simulink model "sm_car_test_ggv_new"  (R2026a)
settings: Solver=ode23t  StopTime=300  MaxStep=0.4  AbsTol=1e-3  EnableMultiTasking=on
PreLoadFcn:
  | % PreLoadFcn Removed for GGV Sweep
PostLoadFcn:
  | % PostLoadFcn Removed for GGV Sweep
InitFcn:
  | sm_car_config_camera;
  | Vehicle = sm_car_vehcfg_checkConfig(Vehicle);
  | sm_car_check_tire_model(bdroot);
StartFcn:
  | tic;
StopFcn:
  | Elapsed_Sim_Time = toc;
  | % disp(['Elapsed Sim Time = ' num2str(Elapsed_Sim_Time)]);
values from neighbouring files (symbols this model uses):
  accel_ramp_rate = 0.1    [sm_car_sweep_ggv_pts.m]
undefined symbols (not defined in the file or in its folder): acc_theta, Axle1D, AxleIn, Camera, Control, drag_frc, Driver, Init, lift_frc, Maneuver, Pedal, Scene, ShaftL1, ShaftL2, ShaftR1, ShaftR2, Visual, X, xy_data_car_side, Y, Z
libraries: sm_lib x270, fl_lib x171, nesl_utility x137, simulink x56, sdl_lib x14, simulink_extras x11, SimscapeFluids_lib x7, Scene_Utilities x6, dspsigops x4, Damper_Element x4, Tire_1x2x x4, ee_lib x3
(part 10 of 20)

== system sm_car_test_ggv_new/World/Scene/Skidpad/Circle Outer L ==
  Solid : sm_lib/Body Elements/Extruded Solid  ExtrusionType=General  PolygonNumSides=3  PolygonOuterRadius=1  PolygonOuterRadiusUnits=m  ExportEntireGeometry=off  ExtrusionCrossSection=xy_data_circ  ExtrusionCrossSectionUnits=m  ExportConvexHullGeometry=off  ExtrusionLength=circ_h  ExtrusionLengthUnits=m  InertiaType=CalculateFromGeometry  BasedOnType=Density  Density=1000  DensityUnits=kg/m^3  Mass=1  MassUnits=kg  CenterOfMass=[0 0 0]  CenterOfMassUnits=m  MomentsOfInertia=[1 1 1]  MomentsOfInertiaUnits=kg*m^2  ProductsOfInertia=[1 1 1]  ProductsOfInertiaUnits=kg*m^2  GraphicType=FromGeometry  MarkerShape=Sphere  MarkerSize=10  GraphicVisPropType=SimpleVisualProperties  GraphicDiffuseColor=[1.0 1.0 0.8]  GraphicOpacity=1.0  GraphicSpecularColor=[0.5 0.5 0.5 1.0]  GraphicAmbientColor=[0.15 0.15 0.15 1.0]  GraphicEmissiveColor=[0.0 0.0 0.0 1.0]  GraphicShininess=75  DoExposeReferenceFrame=on  SerializedFrames=<Frames/>
  W : PMIOPort  Side=Right
  connections:
  Solid/RConn1 -- W/RConn1

== system sm_car_test_ggv_new/World/Scene/Skidpad/Circle Outer R ==
  Solid : sm_lib/Body Elements/Extruded Solid  ExtrusionType=General  PolygonNumSides=3  PolygonOuterRadius=1  PolygonOuterRadiusUnits=m  ExportEntireGeometry=off  ExtrusionCrossSection=xy_data_circ  ExtrusionCrossSectionUnits=m  ExportConvexHullGeometry=off  ExtrusionLength=circ_h  ExtrusionLengthUnits=m  InertiaType=CalculateFromGeometry  BasedOnType=Density  Density=1000  DensityUnits=kg/m^3  Mass=1  MassUnits=kg  CenterOfMass=[0 0 0]  CenterOfMassUnits=m  MomentsOfInertia=[1 1 1]  MomentsOfInertiaUnits=kg*m^2  ProductsOfInertia=[1 1 1]  ProductsOfInertiaUnits=kg*m^2  GraphicType=FromGeometry  MarkerShape=Sphere  MarkerSize=10  GraphicVisPropType=SimpleVisualProperties  GraphicDiffuseColor=[1.0 1.0 0.8]  GraphicOpacity=1.0  GraphicSpecularColor=[0.5 0.5 0.5 1.0]  GraphicAmbientColor=[0.15 0.15 0.15 1.0]  GraphicEmissiveColor=[0.0 0.0 0.0 1.0]  GraphicShininess=75  DoExposeReferenceFrame=on  SerializedFrames=<Frames/>
  W : PMIOPort  Side=Right
  connections:
  Solid/RConn1 -- W/RConn1

== system sm_car_test_ggv_new/World/Scene/Skidpad/Ground Plane ==
  Floor : sm_lib/Body Elements/Brick Solid  BrickDimensions=[gp_l, gp_w, gp_h]  BrickDimensionsUnits=m  ExportEntireGeometry=off  InertiaType=CalculateFromGeometry  BasedOnType=Density  Density=1000  DensityUnits=kg/m^3  Mass=1  MassUnits=kg  CenterOfMass=[0 0 0]  CenterOfMassUnits=m  MomentsOfInertia=[1 1 1]  MomentsOfInertiaUnits=kg*m^2  ProductsOfInertia=[0 0 0]  ProductsOfInertiaUnits=kg*m^2  GraphicType=FromGeometry  MarkerShape=Sphere  MarkerSize=10  GraphicVisPropType=SimpleVisualProperties  GraphicDiffuseColor=gp_clr  GraphicOpacity=gp_opc  GraphicSpecularColor=[0.5 0.5 0.5 1.0]  GraphicAmbientColor=[0.15 0.15 0.15 1.0]  GraphicEmissiveColor=[0.0 0.0 0.0 1.0]  GraphicShininess=75  DoExposeReferenceFrame=off  SerializedFrames=<Frames><Frame><Id>Frame1</Id><Value><Name>F</Name><Origin><Source>GeometricFeature</Source><FeatureName>+z surface</FeatureName></Origin><PrimaryAxis><DefinedDirection>+Z</DefinedDirection><Source>ReferenceFrame</Source><SourceDirection>+Z</SourceDirection><FeatureName></FeatureName></PrimaryAxis><SecondaryAxis><DefinedDirection>+X</DefinedDirection><Source>ReferenceFrame</Source><SourceDirection>+X</SourceDirection><FeatureName></FeatureName></SecondaryAxis></Value></Frame></Frames>
  W : PMIOPort  Side=Right
  connections:
  Floor/LConn1 -- W/RConn1

== system sm_car_test_ggv_new/Controller/Default/State Estimation/Sensor Noise Simulation/noise COG ==
  <vx> : Inport
  <COG> : Inport  Port=2
  Add1 : Sum
  Add2 : Sum
  Band-Limited White Noise1 : simulink/Sources/Band-Limited White Noise  Cov=[7e-3]  Ts=0.1  seed=[08854]
  Band-Limited White Noise2 : simulink/Sources/Band-Limited White Noise  Cov=[1.2e-5]  Ts=0.1  seed=[08854]
  Compare To Constant : simulink/Logic and Bit Operations/Compare To Constant  relop=<=  const=0.15  OutDataTypeStr=boolean
  Quantizer1 : Quantizer  QuantizationInterval=deg2rad(0.1)
  Quantizer2 : Quantizer  QuantizationInterval=deg2rad(0.1)
  Switch : Switch  Criteria=u2 ~= 0  SaturateOnIntegerOverflow=off  InputSameDT=off
  Zero-Order Hold1 : ZeroOrderHold  SampleTime=0.1
  Zero-Order Hold2 : ZeroOrderHold  SampleTime=0.1
  COG_n : Outport
  wires:
  Add2/1 -> Switch/3  "COG_n"
  <COG>/1 -> Quantizer1/1, Quantizer2/1
  Zero-Order Hold2/1 -> Add2/1
  Band-Limited White Noise2/1 -> Add2/2
  Quantizer2/1 -> Zero-Order Hold2/1
  <vx>/1 -> Compare To Constant/1
  Compare To Constant/1 -> Switch/2
  Quantizer1/1 -> Zero-Order Hold1/1
  Band-Limited White Noise1/1 -> Add1/2
  Zero-Order Hold1/1 -> Add1/1
  Add1/1 -> Switch/1  "COG_n"
  Switch/1 -> COG_n/1

== system sm_car_test_ggv_new/Controller/Default/State Estimation/Sensor Noise Simulation/noise a_x ==
  <w> : Inport
  Add2 : Sum
  Band-Limited White Noise2 : simulink/Sources/Band-Limited White Noise  Cov=[0.0024]  Ts=0.01  seed=[512361]
  Quantizer2 : Quantizer  QuantizationInterval=0.0047
  Zero-Order Hold2 : ZeroOrderHold  SampleTime=0.01
  a_x_n : Outport
  wires:
  Add2/1 -> a_x_n/1  "a_x_n"
  <w>/1 -> Quantizer2/1
  Zero-Order Hold2/1 -> Add2/1
  Band-Limited White Noise2/1 -> Add2/2
  Quantizer2/1 -> Zero-Order Hold2/1

== system sm_car_test_ggv_new/Controller/Default/State Estimation/Sensor Noise Simulation/noise a_y ==
  <w> : Inport
  Add2 : Sum
  Band-Limited White Noise2 : simulink/Sources/Band-Limited White Noise  Cov=[0.0024]  Ts=0.01  seed=[092756]
  Quantizer2 : Quantizer  QuantizationInterval=0.0047
  Zero-Order Hold2 : ZeroOrderHold  SampleTime=0.01
  a_y_n : Outport
  wires:
  Add2/1 -> a_y_n/1  "a_y_n"
  <w>/1 -> Quantizer2/1
  Zero-Order Hold2/1 -> Add2/1
  Band-Limited White Noise2/1 -> Add2/2
  Quantizer2/1 -> Zero-Order Hold2/1

== system sm_car_test_ggv_new/Controller/Default/State Estimation/Sensor Noise Simulation/noise omega_fl ==
  <w> : Inport
  Add2 : Sum
  Band-Limited White Noise2 : simulink/Sources/Band-Limited White Noise  Cov=[1e-4]  Ts=0.01  seed=[12451]
  Quantizer2 : Quantizer  QuantizationInterval=2 * pi / 25
  Zero-Order Hold2 : ZeroOrderHold  SampleTime=0.01
  omega_rl : Outport
  wires:
  Add2/1 -> omega_rl/1  "omega_rl"
  <w>/1 -> Quantizer2/1
  Zero-Order Hold2/1 -> Add2/1
  Band-Limited White Noise2/1 -> Add2/2
  Quantizer2/1 -> Zero-Order Hold2/1

== system sm_car_test_ggv_new/Controller/Default/State Estimation/Sensor Noise Simulation/noise omega_fr ==
  <w> : Inport
  Add3 : Sum
  Band-Limited White Noise3 : simulink/Sources/Band-Limited White Noise  Cov=[1e-4]  Ts=0.01  seed=[68595]
  Quantizer3 : Quantizer  QuantizationInterval=2 * pi / 25
  Zero-Order Hold3 : ZeroOrderHold  SampleTime=0.01
  omega_rr : Outport
  wires:
  Add3/1 -> omega_rr/1  "omega_rr"
  Band-Limited White Noise3/1 -> Add3/2
  Zero-Order Hold3/1 -> Add3/1
  <w>/1 -> Quantizer3/1
  Quantizer3/1 -> Zero-Order Hold3/1

== system sm_car_test_ggv_new/Controller/Default/State Estimation/Sensor Noise Simulation/noise omega_rl ==
  <w> : Inport
  Add : Sum
  Band-Limited White Noise : simulink/Sources/Band-Limited White Noise  Cov=[1e-4]  Ts=0.01  seed=[23341]
  Quantizer : Quantizer  QuantizationInterval=2 * pi / 94
  Zero-Order Hold : ZeroOrderHold  SampleTime=0.01
  omega_rl : Outport
  wires:
  Quantizer/1 -> Zero-Order Hold/1
  <w>/1 -> Quantizer/1
  Band-Limited White Noise/1 -> Add/2
  Add/1 -> omega_rl/1  "omega_rl"
  Zero-Order Hold/1 -> Add/1

== system sm_car_test_ggv_new/Controller/Default/State Estimation/Sensor Noise Simulation/noise omega_rr ==
  <w> : Inport
  Add1 : Sum
  Band-Limited White Noise1 : simulink/Sources/Band-Limited White Noise  Cov=[1e-4]  Ts=0.01  seed=[41245]
  Quantizer1 : Quantizer  QuantizationInterval=2 * pi / 94
  Zero-Order Hold1 : ZeroOrderHold  SampleTime=0.01
  omega_rr : Outport
  wires:
  Add1/1 -> omega_rr/1  "omega_rr"
  Quantizer1/1 -> Zero-Order Hold1/1
  <w>/1 -> Quantizer1/1
  Band-Limited White Noise1/1 -> Add1/2
  Zero-Order Hold1/1 -> Add1/1

== system sm_car_test_ggv_new/Controller/Default/State Estimation/Sensor Noise Simulation/noise v_gps ==
  <vz> : Inport
  <vx> : Inport  Port=2
  <vy> : Inport  Port=3
  Add : Sum  Inputs=+++
  Add2 : Sum
  Band-Limited White Noise2 : simulink/Sources/Band-Limited White Noise  Cov=[9e-4]  Ts=0.1  seed=[645743]
  Quantizer2 : Quantizer  QuantizationInterval=0.01
  Sqrt : Sqrt
  Square : Math  Operator=square
  Square1 : Math  Operator=square
  Square2 : Math  Operator=square
  Zero-Order Hold2 : ZeroOrderHold  SampleTime=0.1
  V_GPS_n : Outport
  wires:
  Quantizer2/1 -> Zero-Order Hold2/1
  Band-Limited White Noise2/1 -> Add2/2
  Zero-Order Hold2/1 -> Add2/1
  Sqrt/1 -> Quantizer2/1
  Add2/1 -> V_GPS_n/1  "V_GPS_n"
  <vz>/1 -> Square/1
  <vx>/1 -> Square1/1
  <vy>/1 -> Square2/1
  Add/1 -> Sqrt/1
  Square/1 -> Add/1
  Square1/1 -> Add/2
  Square2/1 -> Add/3

== system sm_car_test_ggv_new/Controller/Default/State Estimation/Sensor Noise Simulation/noise yaw ==
  <w> : Inport
  Add2 : Sum
  Band-Limited White Noise2 : simulink/Sources/Band-Limited White Noise  Cov=[1.2e-7]  Ts=0.01  seed=[211845]
  Quantizer2 : Quantizer  QuantizationInterval=deg2rad(0.1)
  Zero-Order Hold2 : ZeroOrderHold  SampleTime=0.01
  aYaw_n : Outport
  wires:
  Quantizer2/1 -> Zero-Order Hold2/1
  Band-Limited White Noise2/1 -> Add2/2
  Zero-Order Hold2/1 -> Add2/1
  <w>/1 -> Quantizer2/1
  Add2/1 -> aYaw_n/1  "aYaw_n"

== system sm_car_test_ggv_new/Controller/Default/State Estimation/Sensor Noise Simulation/noise yaw rate ==
  <w> : Inport
  Add2 : Sum
  Band-Limited White Noise2 : simulink/Sources/Band-Limited White Noise  Cov=[7.6e-7]  Ts=0.01  seed=[809953]
  Quantizer2 : Quantizer  QuantizationInterval=0.001
  Zero-Order Hold2 : ZeroOrderHold  SampleTime=0.01
  nYaw_n : Outport
  wires:
  Quantizer2/1 -> Zero-Order Hold2/1
  Band-Limited White Noise2/1 -> Add2/2
  Zero-Order Hold2/1 -> Add2/1
  <w>/1 -> Quantizer2/1
  Add2/1 -> nYaw_n/1  "nYaw_n"

== system sm_car_test_ggv_new/Controller/TrqVec 4Motor/Brake Control/ABS/Calculate Slip ==
  WhlSpd : Inport
  VehSpdEst : Inport  Port=2
  Abs : Abs  ZeroCross=off  SaturateOnIntegerOverflow=off
  Bus Creator : BusCreator  Inputs=4
  Bus Selector1 : BusSelector  OutputSignals=L1.v,R1.v,L2.v,R2.v
  Constant : Constant
  Demux : Demux
  Fcn{,1..3} (4 alike) : Fcn  Expr=abs(u(1)*u(2)-u(3))/u(3)
  Mux{,1..3} (4 alike) : Mux  Inputs=3
  Mux4 : Mux
  Mux5 : Mux
  Product : Product
  Saturation : Saturate  UpperLimit=inf  LowerLimit=eps  ZeroCross=off
  Saturation1 : Saturate  UpperLimit=1  LowerLimit=0
  Sign : Signum  ZeroCross=off
  Wheel Speeds and Slip : Scope  NumInputPorts=2
      settings: ActiveDisplayYMinimum=-11.64241  ActiveDisplayYMaximum=114.01232  DataLoggingVariableName=ScopeData2
  Slip : Outport  VectorParamsAs1DForOutWhenUnconnected=off
  wires:
  WhlSpd/1 -> Bus Selector1/1
  Bus Selector1/2 -> Mux4/2, Mux1/2  "<v>"
  Bus Selector1/4 -> Mux4/4, Mux3/2  "<v>"
  Bus Selector1/1 -> Mux4/1, Mux/2  "<v>"
  Bus Selector1/3 -> Mux4/3, Mux2/2  "<v>"
  Constant/1 -> Mux/1, Mux1/1, Mux3/1, Mux2/1
  VehSpdEst/1 -> Sign/1, Abs/1
  Demux/1 -> Bus Creator/1  "L1"
  Demux/2 -> Bus Creator/2  "R1"
  Demux/3 -> Bus Creator/3  "L2"
  Demux/4 -> Bus Creator/4  "R2"
  Bus Creator/1 -> Wheel Speeds and Slip/2, Slip/1  "Slip"
  Product/1 -> Mux3/3, Mux2/3, Mux1/3, Mux/3
  Abs/1 -> Saturation/1
  Saturation/1 -> Product/1
  Sign/1 -> Product/2
  Mux/1 -> Fcn/1
  Mux1/1 -> Fcn1/1
  Mux2/1 -> Fcn2/1
  Mux3/1 -> Fcn3/1
  Mux4/1 -> Wheel Speeds and Slip/1  "Wheel Speeds"
  Mux5/1 -> Saturation1/1
  Saturation1/1 -> Demux/1
  Fcn/1 -> Mux5/1  "L1"
  Fcn1/1 -> Mux5/2  "R1"
  Fcn2/1 -> Mux5/3  "L2"
  Fcn3/1 -> Mux5/4  "R2"

== system sm_car_test_ggv_new/Controller/TrqVec 4Motor/Brake Control/ABS/Sensor ==
  Body : Inport
  WhlSpd : Inport  Port=2
  Bus Creator{,3..5} (4 alike) : BusCreator  Inputs=1
  Bus Creator6 : BusCreator  Inputs=5
  Bus Selector : BusSelector  OutputSignals=vx,vy  OutputAsBus=on
  Bus Selector4 : BusSelector  OutputSignals=WhlL1.n,WhlR1.n,WhlL2.n,WhlR2.n,WhlL2.qxyz
  Gain : Gain  Gain=3.6*abs_tire_radiusF
  Gain1 : Gain  Gain=3.6*abs_tire_radiusF
  Gain2 : Gain  Gain=3.6*abs_tire_radiusR
  Gain3 : Gain  Gain=3.6*abs_tire_radiusR
  Gain4 : Gain  Gain=3.6
  Terminator1 : Terminator  Commented=on
  Vel in xy plane : Fcn  Expr=sqrt(u(1)^2+u(2)^2)
  missing tooth : Subsystem  Commented=on
  GroundSpd : Outport  VectorParamsAs1DForOutWhenUnconnected=off
  wires:
  Gain1/1 -> Bus Creator3/1  "v"
  missing tooth/1(Out1) -> Terminator1/1  "v"
  Gain2/1 -> Bus Creator4/1  "v"
  Bus Selector4/5 -> missing tooth/2(<qxyz>)  "<qxyz>"
  Bus Creator5/1 -> Bus Creator6/5  "R2"
  Gain3/1 -> Bus Creator5/1  "v"
  Bus Creator/1 -> Bus Creator6/2  "L1"
  Bus Selector4/2 -> Gain1/1  "<n>"
  Bus Creator4/1 -> Bus Creator6/4  "L2"
  Bus Selector4/3 -> Gain2/1, missing tooth/1(<omega>)  "<n>"
  Gain/1 -> Bus Creator/1  "v"
  Body/1 -> Bus Selector/1
  Bus Creator3/1 -> Bus Creator6/3  "R1"
  Gain4/1 -> Bus Creator6/1  "v"
  Bus Selector4/1 -> Gain/1  "<n>"
  Bus Selector4/4 -> Gain3/1  "<n>"
  WhlSpd/1 -> Bus Selector4/1
  Bus Creator6/1 -> GroundSpd/1
  Vel in xy plane/1 -> Gain4/1  "speed"
  Bus Selector/1 -> Vel in xy plane/1

== system sm_car_test_ggv_new/Controller/TrqVec 4Motor/Brake Control/ABS/Valve Control L1 ==
  Slip : Inport
  vSpdEst : Inport  Port=2
  Categorize Surface : Subsystem
  Code to Valves : Subsystem
  Demux : Demux  Outputs=2
  Logic : Stateflow chart  TreatAsAtomicUnit=on
  Mux : Mux  Inputs=2
  Product : Product
  Subsystem : Subsystem
  Subsystem1 : Subsystem
  Valve : Outport  VectorParamsAs1DForOutWhenUnconnected=off
  wires:
  Logic/1(Mod_State) -> Categorize Surface/1(Mod State), Code to Valves/1(C)
  Logic/2(Mod_Dur) -> Product/2
  Slip/1 -> Logic/1(Slip)
  Code to Valves/1(V) -> Product/1
  vSpdEst/1 -> Logic/2(vSpdEst)
  Product/1 -> Demux/1
  Demux/1 -> Subsystem/1(OnT)
  Demux/2 -> Subsystem1/1(OnT)
  Mux/1 -> Valve/1
  Subsystem/1(vSig) -> Mux/1, Categorize Surface/2(Apply Valve)
  Subsystem1/1(vSig) -> Mux/2

== system sm_car_test_ggv_new/Controller/TrqVec 4Motor/Brake Control/ABS/Valve Control L2 ==
  Slip : Inport
  vSpdEst : Inport  Port=2
  Categorize Surface : Subsystem
  Code to Valves : Subsystem
  Demux : Demux  Outputs=2
  Logic : Stateflow chart  TreatAsAtomicUnit=on
  Mux : Mux  Inputs=2
  Product : Product
  Subsystem : Subsystem
  Subsystem1 : Subsystem
  Valve : Outport  VectorParamsAs1DForOutWhenUnconnected=off
  wires:
  Logic/1(Mod_State) -> Categorize Surface/1(Mod State), Code to Valves/1(C)
  Logic/2(Mod_Dur) -> Product/2
  Slip/1 -> Logic/1(Slip)
  Code to Valves/1(V) -> Product/1
  vSpdEst/1 -> Logic/2(vSpdEst)
  Product/1 -> Demux/1
  Demux/1 -> Subsystem/1(OnT)
  Demux/2 -> Subsystem1/1(OnT)
  Mux/1 -> Valve/1
  Subsystem/1(vSig) -> Mux/1, Categorize Surface/2(Apply Valve)
  Subsystem1/1(vSig) -> Mux/2

== system sm_car_test_ggv_new/Controller/TrqVec 4Motor/Brake Control/ABS/Valve Control R1 ==
  Slip : Inport
  vSpdEst : Inport  Port=2
  Categorize Surface : Subsystem
  Code to Valves : Subsystem
  Demux : Demux  Outputs=2
  Logic : Stateflow chart  TreatAsAtomicUnit=on
  Mux : Mux  Inputs=2
  Product : Product
  Subsystem : Subsystem
  Subsystem1 : Subsystem
  Valve : Outport  VectorParamsAs1DForOutWhenUnconnected=off
  wires:
  Logic/1(Mod_State) -> Categorize Surface/1(Mod State), Code to Valves/1(C)
  Logic/2(Mod_Dur) -> Product/2
  Slip/1 -> Logic/1(Slip)
  Code to Valves/1(V) -> Product/1
  vSpdEst/1 -> Logic/2(vSpdEst)
  Product/1 -> Demux/1
  Demux/1 -> Subsystem/1(OnT)
  Demux/2 -> Subsystem1/1(OnT)
  Mux/1 -> Valve/1
  Subsystem/1(vSig) -> Mux/1, Categorize Surface/2(Apply Valve)
  Subsystem1/1(vSig) -> Mux/2

== system sm_car_test_ggv_new/Controller/TrqVec 4Motor/Brake Control/ABS/Valve Control R2 ==
  Slip : Inport
  vSpdEst : Inport  Port=2
  Categorize Surface : Subsystem
  Code to Valves : Subsystem
  Demux : Demux  Outputs=2
  Logic : Stateflow chart  TreatAsAtomicUnit=on
  Mux : Mux  Inputs=2
  Product : Product
  Subsystem : Subsystem
  Subsystem1 : Subsystem
  Valve : Outport  VectorParamsAs1DForOutWhenUnconnected=off
  wires:
  Logic/1(Mod_State) -> Categorize Surface/1(Mod State), Code to Valves/1(C)
  Logic/2(Mod_Dur) -> Product/2
  Slip/1 -> Logic/1(Slip)
  Code to Valves/1(V) -> Product/1
  vSpdEst/1 -> Logic/2(vSpdEst)
  Product/1 -> Demux/1
  Demux/1 -> Subsystem/1(OnT)
  Demux/2 -> Subsystem1/1(OnT)
  Mux/1 -> Valve/1
  Subsystem/1(vSig) -> Mux/1, Categorize Surface/2(Apply Valve)
  Subsystem1/1(vSig) -> Mux/2

== system sm_car_test_ggv_new/Controller/TrqVec 4Motor/Brake Control/ABS/Vehicle Speed ==
  Sensors : Inport
  Bus Selector : BusSelector  OutputSignals=v
  vSpdEst : Outport  VectorParamsAs1DForOutWhenUnconnected=off
  wires:
  Sensors/1 -> Bus Selector/1
  Bus Selector/1 -> vSpdEst/1  "<v>"

== system sm_car_test_ggv_new/Controller/TrqVec 4Motor/Power_TqVec/Torque Vectoring/Accel Torque Request ==
  note: Assumes both rear motors have same torque speed curve
  MotSpdL2 : Inport
  MotSpdR2 : Inport  Port=2
  MaxMotTrqVsSpdA1 : Lookup_n-D  NumberOfTableDimensions=1  BreakpointsForDimension1=Control.MotorL2.TorqueSpd.w.Value  Table=Control.MotorL2.TorqueSpd.trq.Value  ExtrapMethod=Clip  UseLastTableValue=on  InternalRulePriority=Speed  OutDataTypeStr=Inherit: Inherit from 'Table data'  RndMeth=Simplest
  Terminator : Terminator
  rads_to_rpm : Gain  Gain=30/pi
  rads_to_rpm1 : Gain  Gain=30/pi
  TrqMax : Outport  VectorParamsAs1DForOutWhenUnconnected=off
  wires:
  rads_to_rpm1/1 -> Terminator/1
  MotSpdR2/1 -> rads_to_rpm1/1
  MaxMotTrqVsSpdA1/1 -> TrqMax/1
  MotSpdL2/1 -> rads_to_rpm/1
  rads_to_rpm/1 -> MaxMotTrqVsSpdA1/1

== system sm_car_test_ggv_new/Controller/TrqVec 4Motor/Power_TqVec/Torque Vectoring/Enable ==
  note: Ramp up amount of torque vectoring over a range.
  note: Steer angle threshold to enable torque vectoring
  vx : Inport
  aSteerWheel : Inport  Port=2
  Abs : Abs  ZeroCross=off  SaturateOnIntegerOverflow=off
  Data Type Conversion : DataTypeConversion  OutDataTypeStr=double  SaturateOnIntegerOverflow=off  RndMeth=Floor
  Divide : Product  Inputs=*/
  Enable vx : simulink/Logic and Bit Operations/Compare To Constant  relop=>  const=vx_enable  OutDataTypeStr=boolean  ZeroCross=off
  Gain : Gain  Gain=0.25
  Product : Product
  Saturation : Saturate  UpperLimit=1  LowerLimit=0  ZeroCross=off
  Subtract : Sum  Inputs=+-
  const : Constant  Value=aSteerWheel_enable
  Enable : Outport  VectorParamsAs1DForOutWhenUnconnected=off
  wires:
  Gain/1 -> Divide/1
  Product/1 -> Enable/1
  Divide/1 -> Saturation/1
  Subtract/1 -> Gain/1
  Abs/1 -> Subtract/1
  Saturation/1 -> Product/2
  Data Type Conversion/1 -> Product/1
  Enable vx/1 -> Data Type Conversion/1
  const/1 -> Subtract/2, Divide/2
  aSteerWheel/1 -> Abs/1
  vx/1 -> Enable vx/1

== system sm_car_test_ggv_new/Controller/TrqVec 4Motor/Power_TqVec/Torque Vectoring/Vehicle Slip Angle Error ==
  vx : Inport
  aSteerWheel : Inport  Port=2
  nYaw : Inport  Port=3
  Add1 : Sum  Inputs=-+
  Distance Yaw Ctr Front Axle : Constant  Value=Vehicle.Chassis.Body.sAxle2.Value(1)/(-2)
  Divide3 : Product  Inputs=*/
  Multiply2 : Product
  Mux : Mux  Inputs=2
  Scope : Scope  NumInputPorts=2
      settings: ActiveDisplayYMinimum=-0.04829  ActiveDisplayYMaximum=0.00545
  Steering Wheel to Driving Wheel : Gain  Gain=aStr_to_aWhl
  Error : Outport  VectorParamsAs1DForOutWhenUnconnected=off
  wires:
  Mux/1 -> Scope/1
  Multiply2/1 -> Divide3/1
  Steering Wheel to Driving Wheel/1 -> Mux/2, Add1/2  "Wheel Angle"
  Distance Yaw Ctr Front Axle/1 -> Multiply2/1
  aSteerWheel/1 -> Steering Wheel to Driving Wheel/1
  nYaw/1 -> Multiply2/2
  Add1/1 -> Scope/2, Error/1  "Error"
  vx/1 -> Divide3/2
  Divide3/1 -> Add1/1, Mux/1  "Vehicle Slip Angle"

== system sm_car_test_ggv_new/Controller/TrqVec_FLC_V3/Power Control/UKF State Estimation/Activation Threshold ==
  vx : Inport
  Compare To Constant : simulink/Logic and Bit Operations/Compare To Constant  relop=>=  const=0.4  OutDataTypeStr=boolean
  Rate Transition3 : RateTransition  Deterministic=off  OutPortSampleTime=0.003
  Enable : Outport
  wires:
  vx/1 -> Compare To Constant/1
  Rate Transition3/1 -> Enable/1
  Compare To Constant/1 -> Rate Transition3/1

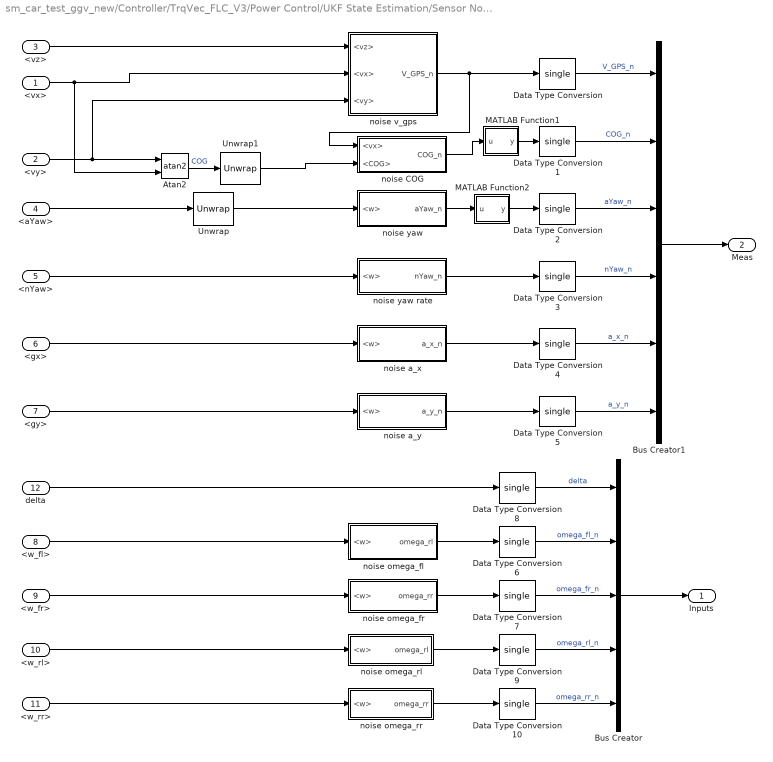
== system sm_car_test_ggv_new/Controller/TrqVec_FLC_V3/Power Control/UKF State Estimation/Sensor Noise Simulation ==
  <vx> : Inport
  <vy> : Inport  Port=2
  <vz> : Inport  Port=3
  <aYaw> : Inport  Port=4
  <nYaw> : Inport  Port=5
  <gx> : Inport  Port=6
  <gy> : Inport  Port=7
  <w_fl> : Inport  Port=8
  <w_fr> : Inport  Port=9
  <w_rl> : Inport  Port=10
  <w_rr> : Inport  Port=11
  delta : Inport  Port=12
  Atan2 : Trigonometry  Operator=atan2
  Bus Creator : BusCreator  Inputs=5
  Bus Creator1 : BusCreator  Inputs=6
  Data Type Conversion{,1..10} (11 alike) : DataTypeConversion  OutDataTypeStr=single  SaturateOnIntegerOverflow=off  RndMeth=Floor
  MATLAB Function1 : MATLAB Function  TreatAsAtomicUnit=on
  MATLAB Function2 : MATLAB Function  TreatAsAtomicUnit=on
  Unwrap : dspsigops/Unwrap  tol=pi  InputProcessing=Columns as channels (frame based)  running=off
  Unwrap1 : dspsigops/Unwrap  tol=pi  InputProcessing=Columns as channels (frame based)  running=off
  noise COG : Subsystem
  noise a_x : Subsystem
  noise a_y : Subsystem
  noise omega_fl : Subsystem
  noise omega_fr : Subsystem
  noise omega_rl : Subsystem
  noise omega_rr : Subsystem
  noise v_gps : Subsystem
  noise yaw : Subsystem
  noise yaw rate : Subsystem
  Inputs : Outport
  Meas : Outport  Port=2
  wires:
  delta/1 -> Data Type Conversion8/1
  <w_fl>/1 -> noise omega_fl/1(<w>)
  <nYaw>/1 -> noise yaw rate/1(<w>)
  <w_fr>/1 -> noise omega_fr/1(<w>)
  <gx>/1 -> noise a_x/1(<w>)
  <aYaw>/1 -> Unwrap/1
  noise a_x/1(a_x_n) -> Data Type Conversion4/1
  noise yaw/1(aYaw_n) -> MATLAB Function2/1(u)
  noise COG/1(COG_n) -> MATLAB Function1/1(u)
  <vx>/1 -> Atan2/2, noise v_gps/2(<vx>)
  noise omega_fl/1(omega_rl) -> Data Type Conversion6/1
  noise a_y/1(a_y_n) -> Data Type Conversion5/1
  Bus Creator/1 -> Inputs/1
  noise omega_rl/1(omega_rl) -> Data Type Conversion9/1
  noise yaw rate/1(nYaw_n) -> Data Type Conversion3/1
  Atan2/1 -> Unwrap1/1  "COG"
  <w_rl>/1 -> noise omega_rl/1(<w>)
  <vy>/1 -> Atan2/1, noise v_gps/3(<vy>)
  <gy>/1 -> noise a_y/1(<w>)
  noise omega_rr/1(omega_rr) -> Data Type Conversion10/1
  <w_rr>/1 -> noise omega_rr/1(<w>)
  noise omega_fr/1(omega_rr) -> Data Type Conversion7/1
  Bus Creator1/1 -> Meas/1
  <vz>/1 -> noise v_gps/1(<vz>)
  Data Type Conversion/1 -> Bus Creator1/1  "V_GPS_n"
  Data Type Conversion1/1 -> Bus Creator1/2  "COG_n"
  Data Type Conversion2/1 -> Bus Creator1/3  "aYaw_n"
  Data Type Conversion3/1 -> Bus Creator1/4  "nYaw_n"
  Data Type Conversion4/1 -> Bus Creator1/5  "a_x_n"
  Data Type Conversion5/1 -> Bus Creator1/6  "a_y_n"
  Data Type Conversion6/1 -> Bus Creator/2  "omega_fl_n"
  Data Type Conversion7/1 -> Bus Creator/3  "omega_fr_n"
  Data Type Conversion8/1 -> Bus Creator/1  "delta"
  Data Type Conversion9/1 -> Bus Creator/4  "omega_rl_n"
  Data Type Conversion10/1 -> Bus Creator/5  "omega_rr_n"
  Unwrap/1 -> noise yaw/1(<w>)
  Unwrap1/1 -> noise COG/2(<COG>)
  noise v_gps/1(V_GPS_n) -> Data Type Conversion/1, noise COG/1(<vx>)
  MATLAB Function1/1(y) -> Data Type Conversion1/1
  MATLAB Function2/1(y) -> Data Type Conversion2/1

== system sm_car_test_ggv_new/Controller/TrqVec_FLC_V3/Power Control/UKF State Estimation/Subsystem ==
  StateTransitionFcnInputs : Inport  PortDimensions=5
  y1 : Inport  Port=2
  Enable : EnablePort
  Adaptive Covariance : MATLAB Function  TreatAsAtomicUnit=on
  Constant : Constant  Value=[0 0 0 0 0]  OutDataTypeStr=single  SampleTime=0.003
  Delay : Delay  DelayLength=1  SampleTime=0.003
  Unscented Kalman Filter : sharedTrackingLibrary/Unscented Kalman Filter  StateTransitionFcn=prediction_model  HasAdditiveProcessNoise=Additive  ProcessNoise=diag([1e-5, 1e-6, 1e-5, 1e-3, 5e-5, 1e-4])  HasTimeVaryingProcessNoise=off  HasStateTransitionFcnExtraArgument=1  InitialState=[0.4; 0; 0; 0; 0; 0]  InitialStateCovariance=diag([0.04, 0.25, 1e-3, 1e-3, 0.1, 0.1])  Alpha=0.1  Beta=2  Kappa=0  MeasurementFcn1=measurement_model  HasMeasurementEnablePort1=off  HasAdditiveMeasurementNoise1=Additive  MeasurementNoise1=diag([1e-3, 1e-6, 5e-4, 1e-4, 1e-2, 1e-2])  HasTimeVaryingMeasurementNoise1=on  HasMeasurementFcnExtraArgument1=1  HasMeasurementWrapping1=on  MeasurementFcn2=myMeasurementFcn  HasMeasurementEnablePort2=off  HasAdditiveMeasurementNoise2=Additive  MeasurementNoise2=1  HasTimeVaryingMeasurementNoise2=off  HasMeasurementFcnExtraArgument2=0  HasMeasurementWrapping2=off  MeasurementFcn3=myMeasurementFcn  HasMeasurementEnablePort3=off  HasAdditiveMeasurementNoise3=Additive  MeasurementNoise3=1  HasTimeVaryingMeasurementNoise3=off  HasMeasurementFcnExtraArgument3=0  HasMeasurementWrapping3=off  MeasurementFcn4=myMeasurementFcn  HasMeasurementEnablePort4=off  HasAdditiveMeasurementNoise4=Additive  MeasurementNoise4=1  HasTimeVaryingMeasurementNoise4=off  HasMeasurementFcnExtraArgument4=0  HasMeasurementWrapping4=off  MeasurementFcn5=myMeasurementFcn  HasMeasurementEnablePort5=off  HasAdditiveMeasurementNoise5=Additive  MeasurementNoise5=1  HasTimeVaryingMeasurementNoise5=off  HasMeasurementFcnExtraArgument5=0  HasMeasurementWrapping5=off  EnableMultirate=off  StateTransitionFcnSampleTime=1  MeasurementFcn1SampleTime=1  MeasurementFcn2SampleTime=1  MeasurementFcn3SampleTime=1  MeasurementFcn4SampleTime=1  MeasurementFcn5SampleTime=1  UseCurrentEstimator=on  OutputStateCovariance=off  DataType=single  SampleTime=0.003  NumberOfMeasurements=1
      settings: LibrarySourceBlock=cstblocks/State Estimation/Unscented Kalman Filter
  xhat : Outport
  wires:
  y1/1 -> Unscented Kalman Filter/2
  Unscented Kalman Filter/1 -> Delay/1, xhat/1
  StateTransitionFcnInputs/1 -> Unscented Kalman Filter/1
  Constant/1 -> Unscented Kalman Filter/4
  Adaptive Covariance/1(R) -> Unscented Kalman Filter/3
  Delay/1 -> Adaptive Covariance/1(xhat)

== system sm_car_test_ggv_new/Driver/Closed Loop/Driver/Lateral Driver/Pure Pursuit ==
  referencePose : Inport
  Distance : Inport  Port=2
  currentPose : Inport  Port=3
  v_x : Inport  Port=4
  Preview : Inport  Port=5
  Direction : Inport  Port=6
  Bus Selector : BusSelector  OutputSignals=pp_preview_x_pts,pp_preview_dist_pts,pp_preview_y_pts,pp_preview_yaw_pts
  Constant : Constant  Value=MAX_STEERING_ANGLE_DEG
  Constant1 : Constant  Value=L_AXLE_DIST
  Constant5 : Constant  Value=LOOKAHEAD_GAIN_KPP
  Constant6 : Constant  Value=MAX_LOOKAHEAD_DIST
  Constant7 : Constant  Value=MIN_LOOKAHEAD_DIST
  Constant8 : Constant  Value=HEADING_WEIGHT_KH
  MATLAB Function1 : MATLAB Function  TreatAsAtomicUnit=on
  Terminator : Terminator
  steeringAngle : Outport
  wires:
  referencePose/1 -> Terminator/1
  v_x/1 -> MATLAB Function1/7(v_x)
  currentPose/1 -> MATLAB Function1/6(currentPose)
  Direction/1 -> MATLAB Function1/8(direction)
  Constant/1 -> MATLAB Function1/10(MAX_STEERING_ANGLE_DEG)
  Constant1/1 -> MATLAB Function1/9(L_AXLE_DIST)
  MATLAB Function1/1(steeringAngle) -> steeringAngle/1
  Constant5/1 -> MATLAB Function1/11(LOOKAHEAD_GAIN_KPP)
  Constant6/1 -> MATLAB Function1/13(MAX_LOOKAHEAD_DIST)
  Constant7/1 -> MATLAB Function1/12(MIN_LOOKAHEAD_DIST)
  Preview/1 -> Bus Selector/1
  Distance/1 -> MATLAB Function1/5(ad_vehicle)
  Bus Selector/1 -> MATLAB Function1/1(pp_preview_x_pts)  "<pp_preview_x_pts>"
  Bus Selector/2 -> MATLAB Function1/2(pp_preview_dist_pts)  "<pp_preview_dist_pts>"
  Bus Selector/3 -> MATLAB Function1/3(pp_preview_y_pts)  "<pp_preview_y_pts>"
  Bus Selector/4 -> MATLAB Function1/4(pp_preview_yaw_pts)  "<pp_preview_yaw_pts>"
  Constant8/1 -> MATLAB Function1/14(HEADING_WEIGHT_KH)

== system sm_car_test_ggv_new/Driver/Closed Loop/Driver/Lateral Driver/Stanley ==
  referencePose : Inport
  Distance : Inport  Port=2
  currentPose : Inport  Port=3
  v_x : Inport  Port=4
  Preview : Inport  Port=5
  Direction : Inport  Port=6
  Constant : Constant  Value=MAX_STEERING_ANGLE_DEG
  Constant1 : Constant  Value=L_AXLE_DIST
  Constant2 : Constant  Value=K_cte_forward
  Constant3 : Constant  Value=K_cte_reverse
  Stanley Driver : MATLAB Function  TreatAsAtomicUnit=on  mask(Lateral Driver (Stanley Driver)){}
      mask help:
      | Implements Stanley method for lateral control.
      | Supports forward and reverse driving.
      | Based on Hoffmann et al. (2007), "Autonomous Automobile Trajectory Tracking for Off-Road Driving"
  Terminator : Terminator
  Terminator1 : Terminator
  steeringAngle : Outport
  wires:
  Distance/1 -> Terminator1/1
  Preview/1 -> Terminator/1
  Stanley Driver/1(steeringAngle) -> steeringAngle/1
  Constant3/1 -> Stanley Driver/8(K_cte_reverse)
  Constant2/1 -> Stanley Driver/7(K_cte_forward)
  Constant1/1 -> Stanley Driver/5(L_AXLE_DIST)
  Constant/1 -> Stanley Driver/6(MAX_STEERING_ANGLE_DEG)
  referencePose/1 -> Stanley Driver/1(referencePose)
  Direction/1 -> Stanley Driver/4(direction)
  currentPose/1 -> Stanley Driver/2(currentPose)
  v_x/1 -> Stanley Driver/3(v_x)

== system sm_car_test_ggv_new/Driver/Closed Loop/Maneuver/Count Lap/Triggered Subsystem ==
  Up Down : Inport
  Trigger : TriggerPort  VariantControl=Variant  ZeroCross=off
  Memory : Memory  InheritSampleTime=on
  Sum : Sum  Inputs=|++
  Num Laps : Outport  VectorParamsAs1DForOutWhenUnconnected=off
  wires:
  Memory/1 -> Sum/1
  Sum/1 -> Memory/1, Num Laps/1
  Up Down/1 -> Sum/2

== system sm_car_test_ggv_new/Driver/Closed Loop/Maneuver/PoseTarget Visual/Pace Car ==
  Left Face : sm_lib/Body Elements/Extruded Solid  ExtrusionType=General  PolygonNumSides=3  PolygonOuterRadius=1  PolygonOuterRadiusUnits=m  ExportEntireGeometry=off  ExtrusionCrossSection=xy_data_car_side  ExtrusionCrossSectionUnits=m  ExportConvexHullGeometry=off  ExtrusionLength=thk_side  ExtrusionLengthUnits=m  InertiaType=PointMass  BasedOnType=Density  Density=1000  DensityUnits=kg/m^3  Mass=0  MassUnits=kg  CenterOfMass=[0 0 0]  CenterOfMassUnits=m  MomentsOfInertia=[1 1 1]  MomentsOfInertiaUnits=kg*m^2  ProductsOfInertia=[0 0 0]  ProductsOfInertiaUnits=kg*m^2  GraphicType=FromGeometry  MarkerShape=Sphere  MarkerSize=10  GraphicVisPropType=SimpleVisualProperties  GraphicDiffuseColor=clr_body_geo_left  GraphicOpacity=opc_body_geo_left  GraphicSpecularColor=[0.5 0.5 0.5 1.0]  GraphicAmbientColor=[0.15 0.15 0.15 1.0]  GraphicEmissiveColor=[0.0 0.0 0.0 1.0]  GraphicShininess=75  DoExposeReferenceFrame=on  SerializedFrames=<Frames/>
  Ornament Front : sm_lib/Body Elements/Extruded Solid  ExtrusionType=General  PolygonNumSides=3  PolygonOuterRadius=1  PolygonOuterRadiusUnits=m  ExportEntireGeometry=off  ExtrusionCrossSection=extr_data_emblem_f  ExtrusionCrossSectionUnits=m  ExportConvexHullGeometry=off  ExtrusionLength=0.01  ExtrusionLengthUnits=m  InertiaType=CalculateFromGeometry  BasedOnType=Density  Density=1000  DensityUnits=kg/m^3  Mass=1  MassUnits=kg  CenterOfMass=[0 0 0]  CenterOfMassUnits=m  MomentsOfInertia=[1 1 1]  MomentsOfInertiaUnits=kg*m^2  ProductsOfInertia=[0 0 0]  ProductsOfInertiaUnits=kg*m^2  GraphicType=FromGeometry  MarkerShape=Sphere  MarkerSize=10  GraphicVisPropType=AdvancedVisualProperties  GraphicDiffuseColor=clr_emblem_f  GraphicOpacity=opc_emblem_f  GraphicSpecularColor=[0.5 0.5 0.5 1.0]  GraphicAmbientColor=[0.15 0.15 0.15 1.0]  GraphicEmissiveColor=[clr_emblem_f 1.0]  GraphicShininess=75  DoExposeReferenceFrame=on  SerializedFrames=<Frames/>
  Ornament Rear : sm_lib/Body Elements/Extruded Solid  ExtrusionType=General  PolygonNumSides=3  PolygonOuterRadius=1  PolygonOuterRadiusUnits=m  ExportEntireGeometry=off  ExtrusionCrossSection=extr_data_emblem_r  ExtrusionCrossSectionUnits=m  ExportConvexHullGeometry=off  ExtrusionLength=0.01  ExtrusionLengthUnits=m  InertiaType=CalculateFromGeometry  BasedOnType=Density  Density=1000  DensityUnits=kg/m^3  Mass=1  MassUnits=kg  CenterOfMass=[0 0 0]  CenterOfMassUnits=m  MomentsOfInertia=[1 1 1]  MomentsOfInertiaUnits=kg*m^2  ProductsOfInertia=[0 0 0]  ProductsOfInertiaUnits=kg*m^2  GraphicType=FromGeometry  MarkerShape=Sphere  MarkerSize=10  GraphicVisPropType=SimpleVisualProperties  GraphicDiffuseColor=clr_emblem_r  GraphicOpacity=opc_emblem_r  GraphicSpecularColor=[0.5 0.5 0.5 1.0]  GraphicAmbientColor=[0.15 0.15 0.15 1.0]  GraphicEmissiveColor=[0.0 0.0 0.0 1.0]  GraphicShininess=75  DoExposeReferenceFrame=on  SerializedFrames=<Frames/>
  Rear View : sm_lib/Frames and Transforms/Reference Frame
  Right Face : sm_lib/Body Elements/Extruded Solid  ExtrusionType=General  PolygonNumSides=3  PolygonOuterRadius=1  PolygonOuterRadiusUnits=m  ExportEntireGeometry=off  ExtrusionCrossSection=xy_data_car_side  ExtrusionCrossSectionUnits=m  ExportConvexHullGeometry=off  ExtrusionLength=thk_side  ExtrusionLengthUnits=m  InertiaType=PointMass  BasedOnType=Density  Density=1000  DensityUnits=kg/m^3  Mass=0  MassUnits=kg  CenterOfMass=[0 0 0]  CenterOfMassUnits=m  MomentsOfInertia=[1 1 1]  MomentsOfInertiaUnits=kg*m^2  ProductsOfInertia=[0 0 0]  ProductsOfInertiaUnits=kg*m^2  GraphicType=FromGeometry  MarkerShape=Sphere  MarkerSize=10  GraphicVisPropType=SimpleVisualProperties  GraphicDiffuseColor=clr_body_geo_right  GraphicOpacity=opc_body_geo_right  GraphicSpecularColor=[0.5 0.5 0.5 1.0]  GraphicAmbientColor=[0.15 0.15 0.15 1.0]  GraphicEmissiveColor=[0.0 0.0 0.0 1.0]  GraphicShininess=75  DoExposeReferenceFrame=on  SerializedFrames=<Frames/>
  Top Surface : sm_lib/Body Elements/Extruded Solid  ExtrusionType=General  PolygonNumSides=3  PolygonOuterRadius=1  PolygonOuterRadiusUnits=m  ExportEntireGeometry=off  ExtrusionCrossSection=xy_data_car_top  ExtrusionCrossSectionUnits=m  ExportConvexHullGeometry=off  ExtrusionLength=car_track  ExtrusionLengthUnits=m  InertiaType=PointMass  BasedOnType=Density  Density=0  DensityUnits=kg/m^3  Mass=0  MassUnits=kg  CenterOfMass=[0 0 0]  CenterOfMassUnits=m  MomentsOfInertia=[1 1 1]  MomentsOfInertiaUnits=kg*m^2  ProductsOfInertia=[0 0 0]  ProductsOfInertiaUnits=kg*m^2  GraphicType=FromGeometry  MarkerShape=Sphere  MarkerSize=10  GraphicVisPropType=SimpleVisualProperties  GraphicDiffuseColor=clr_body_geo_top  GraphicOpacity=opc_body_geo_top  GraphicSpecularColor=[0.5 0.5 0.5 1.0]  GraphicAmbientColor=[0.15 0.15 0.15 1.0]  GraphicEmissiveColor=[0.0 0.0 0.0 1.0]  GraphicShininess=75  DoExposeReferenceFrame=on  SerializedFrames=<Frames/>
  Transform Extrusion Axes : sm_lib/Frames and Transforms/Rigid Transform  RotationMethod=StandardAxis  FollAlignAxisA=+X  BaseAlignAxisA=+Y  FollAlignAxisB=+Y  BaseAlignAxisB=+Z  RotationStandardAxis=+X  RotationAngle=90  RotationAngleUnits=deg  RotationArbitraryAxis=[0 0 1]  RotationSequenceAxes=FollowerAxes  RotationSequence=XYX  RotationSequenceAngles=[0 0 0]  RotationSequenceAnglesUnits=deg  RotationMatrix=[1 0 0; 0 1 0; 0 0 1]  Quaternion=[1 0 0 0]  TranslationMethod=None  TranslationCartesianOffset=[0 0 0]  TranslationCartesianOffsetUnits=m  TranslationStandardAxis=+Z  TranslationStandardOffset=0  TranslationStandardOffsetUnits=m  TranslationROffset=0  TranslationROffsetUnits=m  TranslationThetaOffset=0  TranslationThetaOffsetUnits=deg  TranslationZOffset=0  TranslationZOffsetUnits=m
  Transform Ornament Front : sm_lib/Frames and Transforms/Rigid Transform  RotationMethod=RotationSequence  FollAlignAxisA=+X  BaseAlignAxisA=+Y  FollAlignAxisB=+Y  BaseAlignAxisB=+Z  RotationStandardAxis=+Z  RotationAngle=90  RotationAngleUnits=deg  RotationArbitraryAxis=[0 0 1]  RotationSequenceAxes=FollowerAxes  RotationSequence=ZXY  RotationSequenceAngles=[90 90 0]  RotationSequenceAnglesUnits=deg  RotationMatrix=[1 0 0; 0 1 0; 0 0 1]  Quaternion=[1 0 0 0]  TranslationMethod=Cartesian  TranslationCartesianOffset=[max(xy_data_car_side(:,1)) 0 min(xy_data_car_side(:,2))+0.15]  TranslationCartesianOffsetUnits=m  TranslationStandardAxis=+Z  TranslationStandardOffset=1  TranslationStandardOffsetUnits=m  TranslationROffset=0  TranslationROffsetUnits=m  TranslationThetaOffset=0  TranslationThetaOffsetUnits=deg  TranslationZOffset=0  TranslationZOffsetUnits=m
  Transform Ornament Rear : sm_lib/Frames and Transforms/Rigid Transform  RotationMethod=RotationSequence  FollAlignAxisA=+X  BaseAlignAxisA=+Y  FollAlignAxisB=+Y  BaseAlignAxisB=+Z  RotationStandardAxis=+Z  RotationAngle=90  RotationAngleUnits=deg  RotationArbitraryAxis=[0 0 1]  RotationSequenceAxes=FollowerAxes  RotationSequence=ZXY  RotationSequenceAngles=[90 90 180]  RotationSequenceAnglesUnits=deg  RotationMatrix=[1 0 0; 0 1 0; 0 0 1]  Quaternion=[1 0 0 0]  TranslationMethod=Cartesian  TranslationCartesianOffset=[min(xy_data_car_side(:,1))+0.1 0 min(xy_data_car_side(:,2))+0.15]  TranslationCartesianOffsetUnits=m  TranslationStandardAxis=+Z  TranslationStandardOffset=1  TranslationStandardOffsetUnits=m  TranslationROffset=0  TranslationROffsetUnits=m  TranslationThetaOffset=0  TranslationThetaOffsetUnits=deg  TranslationZOffset=0  TranslationZOffsetUnits=m
  Transform Rear View : sm_lib/Frames and Transforms/Rigid Transform  RotationMethod=None  FollAlignAxisA=+X  BaseAlignAxisA=+Y  FollAlignAxisB=+Y  BaseAlignAxisB=+Z  RotationStandardAxis=+Z  RotationAngle=0.0  RotationAngleUnits=deg  RotationArbitraryAxis=[0 0 1]  RotationSequenceAxes=FollowerAxes  RotationSequence=XYX  RotationSequenceAngles=[0 0 0]  RotationSequenceAnglesUnits=deg  RotationMatrix=[1 0 0; 0 1 0; 0 0 1]  Quaternion=[1 0 0 0]  TranslationMethod=Cartesian  TranslationCartesianOffset=[min(xy_data_car_side(:,1))-4 0 min(xy_data_car_side(:,2))+1]  TranslationCartesianOffsetUnits=m  TranslationStandardAxis=+Z  TranslationStandardOffset=0  TranslationStandardOffsetUnits=m  TranslationROffset=0  TranslationROffsetUnits=m  TranslationThetaOffset=0  TranslationThetaOffsetUnits=deg  TranslationZOffset=0  TranslationZOffsetUnits=m
  Transform Reference : sm_lib/Frames and Transforms/Rigid Transform  RotationMethod=None  FollAlignAxisA=+X  BaseAlignAxisA=+Y  FollAlignAxisB=+Y  BaseAlignAxisB=+Z  RotationStandardAxis=+Z  RotationAngle=0.0  RotationAngleUnits=deg  RotationArbitraryAxis=[0 0 1]  RotationSequenceAxes=FollowerAxes  RotationSequence=XYX  RotationSequenceAngles=[0 0 0]  RotationSequenceAnglesUnits=deg  RotationMatrix=[1 0 0; 0 1 0; 0 0 1]  Quaternion=[1 0 0 0]  TranslationMethod=Cartesian  TranslationCartesianOffset=offset_ref  TranslationCartesianOffsetUnits=m  TranslationStandardAxis=+Z  TranslationStandardOffset=0  TranslationStandardOffsetUnits=m  TranslationROffset=0  TranslationROffsetUnits=m  TranslationThetaOffset=0  TranslationThetaOffsetUnits=deg  TranslationZOffset=0  TranslationZOffsetUnits=m
  Transform Left Face : sm_lib/Frames and Transforms/Rigid Transform  RotationMethod=None  FollAlignAxisA=+X  BaseAlignAxisA=+Y  FollAlignAxisB=+Y  BaseAlignAxisB=+Z  RotationStandardAxis=+Z  RotationAngle=0.0  RotationAngleUnits=deg  RotationArbitraryAxis=[0 0 1]  RotationSequenceAxes=FollowerAxes  RotationSequence=XYX  RotationSequenceAngles=[0 0 0]  RotationSequenceAnglesUnits=deg  RotationMatrix=[1 0 0; 0 1 0; 0 0 1]  Quaternion=[1 0 0 0]  TranslationMethod=StandardAxis  TranslationCartesianOffset=[0 0 0]  TranslationCartesianOffsetUnits=m  TranslationStandardAxis=-Z  TranslationStandardOffset=car_track/2-thk_side/2  TranslationStandardOffsetUnits=m  TranslationROffset=0  TranslationROffsetUnits=m  TranslationThetaOffset=0  TranslationThetaOffsetUnits=deg  TranslationZOffset=0  TranslationZOffsetUnits=m
  Transform Right Face : sm_lib/Frames and Transforms/Rigid Transform  RotationMethod=None  FollAlignAxisA=+X  BaseAlignAxisA=+Y  FollAlignAxisB=+Y  BaseAlignAxisB=+Z  RotationStandardAxis=+Z  RotationAngle=0.0  RotationAngleUnits=deg  RotationArbitraryAxis=[0 0 1]  RotationSequenceAxes=FollowerAxes  RotationSequence=XYX  RotationSequenceAngles=[0 0 0]  RotationSequenceAnglesUnits=deg  RotationMatrix=[1 0 0; 0 1 0; 0 0 1]  Quaternion=[1 0 0 0]  TranslationMethod=StandardAxis  TranslationCartesianOffset=[0 0 0]  TranslationCartesianOffsetUnits=m  TranslationStandardAxis=+Z  TranslationStandardOffset=car_track/2-thk_side/2  TranslationStandardOffsetUnits=m  TranslationROffset=0  TranslationROffsetUnits=m  TranslationThetaOffset=0  TranslationThetaOffsetUnits=deg  TranslationZOffset=0  TranslationZOffsetUnits=m
  FA : PMIOPort  Side=Right
  P : PMIOPort  Port=2  Side=Left
  connections:
  Transform Reference/LConn1 -- P/RConn1 -- FA/RConn1
  Transform Rear View/RConn1 -- Rear View/RConn1
  Transform Reference/RConn1 -- Transform Ornament Front/LConn1 -- Transform Ornament Rear/LConn1 -- Transform Rear View/LConn1 -- Transform Extrusion Axes/LConn1
  Left Face/RConn1 -- Transform Left Face/RConn1
  Transform Extrusion Axes/RConn1 -- Transform Right Face/LConn1 -- Top Surface/RConn1 -- Transform Left Face/LConn1
  Right Face/RConn1 -- Transform Right Face/RConn1
  Transform Ornament Front/RConn1 -- Ornament Front/RConn1
  Transform Ornament Rear/RConn1 -- Ornament Rear/RConn1

== system sm_car_test_ggv_new/Vehicle/Vehicle/Brakes/PedalAbstract DiscDisc/Actuator L1 ==
  Pedal : Inport
  Filter : TransferFcn  Numerator=brk_max_p  Denominator=[brk_filt 1]
  Simulink-PS Converter : nesl_utility/Simulink-PS Converter  PhysicalDomain=network_engine_domain  SubClassName=ps_input  LeftPortType=input  RightPortType=output  PseudoPeriodic=off  Frequencies=[]  NoiseDistribution=none  NoiseParameters=[]  Unit=1  AffineConversion=off  FilteringAndDerivatives=provide  SimscapeFilterOrder=1  InputFilterTimeConstant=0.001  UdotUserProvided=0
  P : PMIOPort  Side=Right
  wires:
  Pedal/1 -> Filter/1
  Filter/1 -> Simulink-PS Converter/1
  connections:
  Simulink-PS Converter/RConn1 -- P/RConn1

== system sm_car_test_ggv_new/Vehicle/Vehicle/Brakes/PedalAbstract DiscDisc/Actuator L2 ==
  Pedal : Inport
  Filter : TransferFcn  Numerator=brk_max_p  Denominator=[brk_filt 1]
  Simulink-PS Converter : nesl_utility/Simulink-PS Converter  PhysicalDomain=network_engine_domain  SubClassName=ps_input  LeftPortType=input  RightPortType=output  PseudoPeriodic=off  Frequencies=[]  NoiseDistribution=none  NoiseParameters=[]  Unit=1  AffineConversion=off  FilteringAndDerivatives=provide  SimscapeFilterOrder=1  InputFilterTimeConstant=0.001  UdotUserProvided=0
  P : PMIOPort  Side=Right
  wires:
  Pedal/1 -> Filter/1
  Filter/1 -> Simulink-PS Converter/1
  connections:
  Simulink-PS Converter/RConn1 -- P/RConn1

== system sm_car_test_ggv_new/Vehicle/Vehicle/Brakes/PedalAbstract DiscDisc/Actuator R1 ==
  Pedal : Inport
  Filter : TransferFcn  Numerator=brk_max_p  Denominator=[brk_filt 1]
  Simulink-PS Converter : nesl_utility/Simulink-PS Converter  PhysicalDomain=network_engine_domain  SubClassName=ps_input  LeftPortType=input  RightPortType=output  PseudoPeriodic=off  Frequencies=[]  NoiseDistribution=none  NoiseParameters=[]  Unit=1  AffineConversion=off  FilteringAndDerivatives=provide  SimscapeFilterOrder=1  InputFilterTimeConstant=0.001  UdotUserProvided=0
  P : PMIOPort  Side=Right
  wires:
  Pedal/1 -> Filter/1
  Filter/1 -> Simulink-PS Converter/1
  connections:
  Simulink-PS Converter/RConn1 -- P/RConn1

== system sm_car_test_ggv_new/Vehicle/Vehicle/Brakes/PedalAbstract DiscDisc/Actuator R2 ==
  Pedal : Inport
  Filter : TransferFcn  Numerator=brk_max_p  Denominator=[brk_filt 1]
  Simulink-PS Converter : nesl_utility/Simulink-PS Converter  PhysicalDomain=network_engine_domain  SubClassName=ps_input  LeftPortType=input  RightPortType=output  PseudoPeriodic=off  Frequencies=[]  NoiseDistribution=none  NoiseParameters=[]  Unit=1  AffineConversion=off  FilteringAndDerivatives=provide  SimscapeFilterOrder=1  InputFilterTimeConstant=0.001  UdotUserProvided=0
  P : PMIOPort  Side=Right
  wires:
  Pedal/1 -> Filter/1
  Filter/1 -> Simulink-PS Converter/1
  connections:
  Simulink-PS Converter/RConn1 -- P/RConn1

== system sm_car_test_ggv_new/Vehicle/Vehicle/Brakes/PedalAbstract DiscDisc/Sensing Torque L1 ==
  Ideal Torque Sensor : fl_lib/Mechanical/Mechanical Sensors/Ideal Torque Sensor
  PS-Simulink Converter : nesl_utility/PS-Simulink Converter  PhysicalDomain=network_engine_domain  SubClassName=ps_output  LeftPortType=input  RightPortType=output  PseudoPeriodic=off  Frequencies=[]  VectorFormat=1-D array  Unit=N*m  AffineConversion=off
  C : PMIOPort  Side=Right
  R : PMIOPort  Port=2  Side=Left
  T : Outport  VectorParamsAs1DForOutWhenUnconnected=off
  wires:
  PS-Simulink Converter/1 -> T/1
  connections:
  PS-Simulink Converter/LConn1 -- Ideal Torque Sensor/RConn2
  Ideal Torque Sensor/RConn1 -- C/RConn1
  Ideal Torque Sensor/LConn1 -- R/RConn1

== system sm_car_test_ggv_new/Vehicle/Vehicle/Brakes/PedalAbstract DiscDisc/Sensing Torque L2 ==
  Ideal Torque Sensor : fl_lib/Mechanical/Mechanical Sensors/Ideal Torque Sensor
  PS-Simulink Converter : nesl_utility/PS-Simulink Converter  PhysicalDomain=network_engine_domain  SubClassName=ps_output  LeftPortType=input  RightPortType=output  PseudoPeriodic=off  Frequencies=[]  VectorFormat=1-D array  Unit=N*m  AffineConversion=off
  C : PMIOPort  Side=Right
  R : PMIOPort  Port=2  Side=Left
  T : Outport  VectorParamsAs1DForOutWhenUnconnected=off
  wires:
  PS-Simulink Converter/1 -> T/1
  connections:
  PS-Simulink Converter/LConn1 -- Ideal Torque Sensor/RConn2
  Ideal Torque Sensor/RConn1 -- C/RConn1
  Ideal Torque Sensor/LConn1 -- R/RConn1

== system sm_car_test_ggv_new/Vehicle/Vehicle/Brakes/PedalAbstract DiscDisc/Sensing Torque R1 ==
  Ideal Torque Sensor : fl_lib/Mechanical/Mechanical Sensors/Ideal Torque Sensor
  PS-Simulink Converter : nesl_utility/PS-Simulink Converter  PhysicalDomain=network_engine_domain  SubClassName=ps_output  LeftPortType=input  RightPortType=output  PseudoPeriodic=off  Frequencies=[]  VectorFormat=1-D array  Unit=N*m  AffineConversion=off
  C : PMIOPort  Side=Right
  R : PMIOPort  Port=2  Side=Left
  T : Outport  VectorParamsAs1DForOutWhenUnconnected=off
  wires:
  PS-Simulink Converter/1 -> T/1
  connections:
  Ideal Torque Sensor/LConn1 -- R/RConn1
  Ideal Torque Sensor/RConn1 -- C/RConn1
  PS-Simulink Converter/LConn1 -- Ideal Torque Sensor/RConn2

== system sm_car_test_ggv_new/Vehicle/Vehicle/Brakes/PedalAbstract DiscDisc/Sensing Torque R2 ==
  Ideal Torque Sensor : fl_lib/Mechanical/Mechanical Sensors/Ideal Torque Sensor
  PS-Simulink Converter : nesl_utility/PS-Simulink Converter  PhysicalDomain=network_engine_domain  SubClassName=ps_output  LeftPortType=input  RightPortType=output  PseudoPeriodic=off  Frequencies=[]  VectorFormat=1-D array  Unit=N*m  AffineConversion=off
  C : PMIOPort  Side=Right
  R : PMIOPort  Port=2  Side=Left
  T : Outport  VectorParamsAs1DForOutWhenUnconnected=off
  wires:
  PS-Simulink Converter/1 -> T/1
  connections:
  Ideal Torque Sensor/LConn1 -- R/RConn1
  Ideal Torque Sensor/RConn1 -- C/RConn1
  PS-Simulink Converter/LConn1 -- Ideal Torque Sensor/RConn2

== system sm_car_test_ggv_new/Vehicle/Vehicle/Chassis/Aero/Subsystem ==
  RdBus : Inport
  Actuator dynamics : Subsystem  mask(First-order lag supporting vector signals){b=0.5, x_initial=0}
      mask prompts: b "Filter time constant"; x_initial "Initial output"
      mask help: Models a lag of the form 1/(b*s+1) where s is the Laplace operator.
  Bus Selector : BusSelector  OutputSignals=fx,fy,fz
  Mux : Mux  Inputs=3
  Simulink-PS Converter : nesl_utility/Simulink-PS Converter  PhysicalDomain=network_engine_domain  SubClassName=ps_input  LeftPortType=input  RightPortType=output  PseudoPeriodic=off  Frequencies=[]  NoiseDistribution=none  NoiseParameters=[]  Unit=1  AffineConversion=off  FilteringAndDerivatives=provide  SimscapeFilterOrder=1  InputFilterTimeConstant=0.001  UdotUserProvided=0
  fWind : PMIOPort  Side=Right
  wires:
  Actuator dynamics/1(Out) -> Simulink-PS Converter/1
  RdBus/1 -> Bus Selector/1
  Bus Selector/3 -> Mux/3  "<fz>"
  Bus Selector/2 -> Mux/2  "<fy>"
  Bus Selector/1 -> Mux/1  "<fx>"
  Mux/1 -> Actuator dynamics/1(In)
  connections:
  Simulink-PS Converter/RConn1 -- fWind/RConn1
